simulink model "[6]DPOS_LLC(Matlab2020a)"  (R2020a)
settings: Solver=VariableStepAuto  StartTime=0.0  StopTime=0.01  RelTol=1e-3
libraries: powerlib x24, commsynccomp2 x1, simulink x1
settings Model: Creator=cr  LastModifiedBy=Yatao
settings DataIOCC: ReturnWorkspaceOutputs=off
settings DebuggingCC: ArithmeticOperatorsInVariantConditions=warning
settings SFSimCC: SimUseLocalCustomCode=off  CustomCodeUndefinedFunction=UseInterfaceOnly
settings RTWCC: RTWUseLocalCustomCode=off
settings CodeAppCC: StateflowObjectComments=on
settings SimscapeCC: SimscapeNormalizeSystem=off

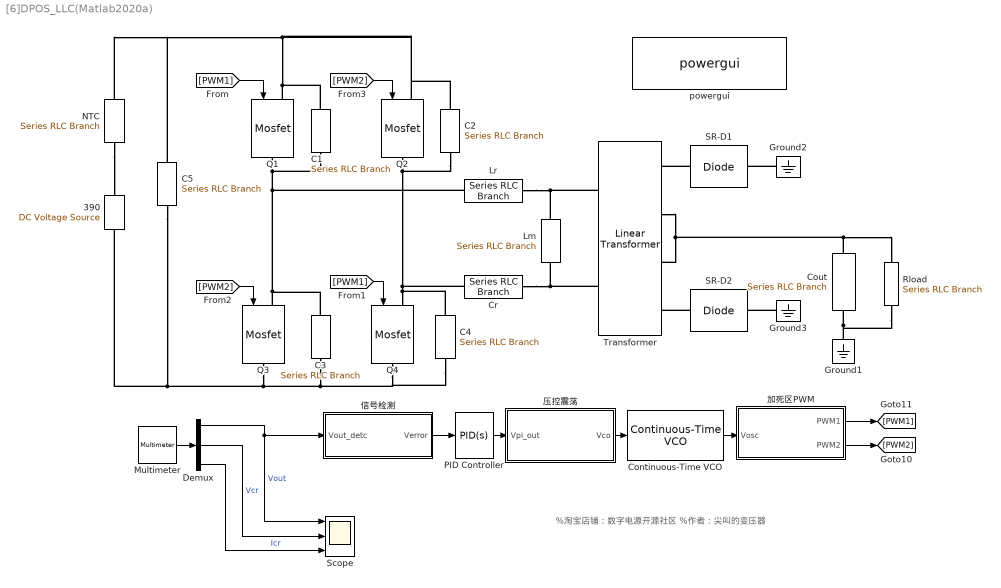
== system [6]DPOS_LLC(Matlab2020a) ==
  note: %淘宝店铺：数字电源开源社区
      | %作者：尖叫的变压器
  " Transformer" : powerlib/Elements/Linear Transformer  UNITS=pu  NominalPower=[ 5000 100e3 ]  winding1=[ 400 0 0 ]  winding2=[ 21 0 0 ]  ThreeWindings=on  winding3=[ 21 0 0 ]  RmLm=[ 1e9 inf ]  Measurements=None  DataType=off
  390 : powerlib/Electrical Sources/DC Voltage Source  Amplitude=390  Measurements=None
  C{1..4} (4 alike) : powerlib/Elements/Series RLC Branch  LConnTagsString=__new0  RConnTagsString=__new0  BranchType=C  Resistance=1  Inductance=1e-3  SetiL0=off  InitialCurrent=0  Capacitance=100e-12  Setx0=off  InitialVoltage=0  Measurements=None
  C5 : powerlib/Elements/Series RLC Branch  LConnTagsString=__new0  RConnTagsString=__new0  BranchType=C  Resistance=1  Inductance=1e-3  SetiL0=off  InitialCurrent=0  Capacitance=100e-6  Setx0=off  InitialVoltage=0  Measurements=None
  Continuous-Time VCO : commsynccomp2/Continuous-Time VCO  Ac=1  Fc=0  Kc=1  Ph=0
      settings: SourceProductBaseCode=CM
  Cout : powerlib/Elements/Series RLC Branch  LConnTagsString=__new0  RConnTagsString=__new0  BranchType=C  Resistance=1  Inductance=1e-3  SetiL0=off  InitialCurrent=0  Capacitance=6000e-6  Setx0=off  InitialVoltage=0  Measurements=None
  Cr : powerlib/Elements/Series RLC Branch  LConnTagsString=__new0  RConnTagsString=__new0  BranchType=C  Resistance=1  Inductance=1e-3  SetiL0=off  InitialCurrent=0  Capacitance=10e-9  Setx0=off  InitialVoltage=0  Measurements=Branch voltage and current
  Demux : Demux  Outputs=3
  Ground1 : powerlib/Elements/Ground  LConnTagsString=a
  Ground2 : powerlib/Elements/Ground  LConnTagsString=a
  Ground3 : powerlib/Elements/Ground  LConnTagsString=a
  Lm : powerlib/Elements/Series RLC Branch  LConnTagsString=__new0  RConnTagsString=__new0  BranchType=L  Resistance=1  Inductance=1500e-6  SetiL0=off  InitialCurrent=0  Capacitance=1e-6  Setx0=off  InitialVoltage=0  Measurements=None
  Lr : powerlib/Elements/Series RLC Branch  LConnTagsString=__new0  RConnTagsString=__new0  BranchType=L  Resistance=1  Inductance=300e-6  SetiL0=off  InitialCurrent=0  Capacitance=1e-6  Setx0=off  InitialVoltage=0  Measurements=None
  Multimeter : powerlib/Measurements/Multimeter  PhasorSimulation=off  OutputType=Complex  sel=[2 1 3]  L=3  Gain=[1 1 1]  yselected={'Ub: Rload','Ub: Cr','Ib: Cr'};  PSBOutputType=1  PSBequivalent=0  AxesSetting=[0,0.1,-100,100]  Display=0  SavedBlockNames=-11
  NTC : powerlib/Elements/Series RLC Branch  LConnTagsString=__new0  RConnTagsString=__new0  BranchType=R  Resistance=1  Inductance=1e-3  SetiL0=off  InitialCurrent=0  Capacitance=100e-12  Setx0=off  InitialVoltage=0  Measurements=None
  PID Controller : simulink/Continuous/PID Controller  Controller=PID  Form=Parallel  TimeDomain=Continuous-time  UseExternalTs=off  SampleTime=-1  IntegratorMethod=Forward Euler  FilterMethod=Forward Euler  ControllerParametersSource=internal  P=0.5  I=0.8  D=2.0  UseFilter=on  N=1  TunerSelectOption=Transfer Function Based (PID Tuner App)  ZeroCross=off  InitialConditionSource=internal  InitialConditionForIntegrator=0  InitialConditionForFilter=0  DifferentiatorICPrevScaledInput=0  ExternalReset=none  TrackingMode=off  Kt=1  LimitOutput=off  UpperSaturationLimit=inf  LowerSaturationLimit=-inf  LinearizeAsGain=on  AntiWindupMode=none  Kb=1  POutMin=[]  POutMax=[]  IOutMin=[]  IOutMax=[]  DOutMin=[]  DOutMax=[]  NOutMin=[]  NOutMax=[]  SumOutMin=[]  SumOutMax=[]  SaturationOutMin=[]  SaturationOutMax=[]  PParamMin=[]  PParamMax=[]  IParamMin=[]  IParamMax=[]  DParamMin=[]  DParamMax=[]  NParamMin=[]  NParamMax=[]  KbParamMin=[]  KbParamMax=[]  KtParamMin=[]  KtParamMax=[]  KbOutMin=[]  KbOutMax=[]  KtOutMin=[]  KtOutMax=[]  IntegratorOutMin=[]  IntegratorOutMax=[]  FilterOutMin=[]  FilterOutMax=[]  SumI1OutMin=[]  SumI1OutMax=[]  SumI2OutMin=[]  SumI2OutMax=[]  SumI3OutMin=[]  SumI3OutMax=[]  SumI4OutMin=[]  SumI4OutMax=[]  SumDOutMin=[]  SumDOutMax=[]  DifferentiatorOutMin=[]  DifferentiatorOutMax=[]  FilterDiffOutCoefMin=[]  FilterDiffOutCoefMax=[]  ReciprocalOutMin=[]  ReciprocalOutMax=[]  SumDenOutMin=[]  SumDenOutMax=[]  SumNumOutMin=[]  SumNumOutMax=[]  DivideOutMin=[]  DivideOutMax=[]  UdiffTsProdOutMin=[]  UdiffTsProdOutMax=[]  NTsProdOutMin=[]  NTsProdOutMax=[]  UintegralTsProdOutMin=[]  UintegralTsProdOutMax=[]  UngainTsProdOutMin=[]  UngainTsProdOutMax=[]  IntegratorContinuousStateAttributes=''  IntegratorStateMustResolveToSignalObject=off  IntegratorRTWStateStorageClass=Auto  FilterContinuousStateAttributes=''  FilterStateMustResolveToSignalObject=off  FilterRTWStateStorageClass=Auto  ParallelPVariant=InternalParameters  IdealPVariant=Disabled  IVariant=InternalParameters  DVariant=InternalParameters  IntegratorVariant=Continuous  SatVariant=Disabled  AWVariant=Passthrough  PCopyVariant=Disabled  TRVariant=Disabled  FdbkBlocksVariant=Forward  IdealPFdbkVariant=Disabled  SatFdbkVariant=Disabled  DerivativeFilterVariant=ContFilter  NVariant=InternalParameters  NCopyVariant=Disabled  FilterICVariant=InternalICsFilter  IntegratorICVariant=InternalICs  ExternalResetVariant=Disabled  TRSumVariant=Passthrough  SumFdbkVariant=Disabled  SumVariant=Sum_PID  TsampFilterVariant=InternalTs  TsampNgainVariant=Passthrough  TsampIntegralVariant=Passthrough
  Q{1..4} (4 alike) : powerlib/Power Electronics/Mosfet  Ron=0.1  Lon=0  Rd=0.07  Vfd=0  IC=0  Rs=1e9  Cs=inf  Measurements=off
  Rload : powerlib/Elements/Series RLC Branch  LConnTagsString=__new0  RConnTagsString=__new0  BranchType=R  Resistance=5  Inductance=1e-3  SetiL0=off  InitialCurrent=0  Capacitance=1e-6  Setx0=off  InitialVoltage=0  Measurements=Branch voltage
  SR-D1 : powerlib/Power Electronics/Diode  Ron=0.001  Lon=0  Vf=0.7  IC=0  UseSnubber=off  Rs=5e9  Cs=10e-12  Measurements=off
  SR-D2 : powerlib/Power Electronics/Diode  Ron=0.001  Lon=0  Vf=0.7  IC=0  UseSnubber=off  Rs=5e9  Cs=10e-12  Measurements=off
  Scope : Scope  NumInputPorts=3
  powergui : powerlib/powergui  Priority=1  SimulationMode=Discrete  SampleTime=1e-8  frequency=60  Iterations=50  frequencyindice=0  Pbase=100e6  ErrMax=1e-4  UnitsV=kV  UnitsW=MW  buscounter=0  FunctionMessages=off  echomessages=off  EnableUseOfTLC=off  CurrentSourceSwitches=off  DisableSnubberDevices=off  DisableRonSwitches=off  DisableVfSwitches=off  DisplayEquations=off  AutomaticDiscreteSolvers=off  SolverType=Tustin/Backward Euler (TBE)  Interpol=off  ExternalGateDelay=off  methode=off  Ts=10  x0status=blocks  SPID=off  SwTol=0  HookPort=off  NonlinearTolerance=1e-4  nMaxIteration=100  ContinueOnMaxIteration=off  RestoreLinks=warning  ResistiveCurrentMeasurement=off  Frange=[0:2:500]  Ylog=off  Xlog=on  ShowGrid=off  save=off  variable=ZData  structure=0  ZoomFFT=off  StartTime=0.0  cycles=1  DisplayStyle=1  fundamental=60  FreqAxis=off  MaxFrequency=1000  frequencyindicesteady=1  RmsSteady=1  display=off
  信号检测 : MATLAB Function  TreatAsAtomicUnit=on
  加死区PWM : MATLAB Function  TreatAsAtomicUnit=on
  压控震荡 : MATLAB Function  TreatAsAtomicUnit=on
  wires:
  [PWM1] -> Q1/1
  [PWM1] -> Q4/1
  [PWM2] -> Q3/1
  [PWM2] -> Q2/1
  信号检测/1(Verror) -> PID Controller/1
  Continuous-Time VCO/1 -> 加死区PWM/1(Vosc)
  加死区PWM/1(PWM1) -> [PWM1]
  加死区PWM/2(PWM2) -> [PWM2]
  压控震荡/1(Vco) -> Continuous-Time VCO/1
  PID Controller/1 -> 压控震荡/1(Vpi_out)
  Multimeter/1 -> Demux/1
  Demux/1 -> Scope/1, 信号检测/1(Vout_detc)  "Vout"
  Demux/2 -> Scope/2  "Vcr"
  Demux/3 -> Scope/3  "Icr"
  connections:
  C3/RConn1 -- C4/RConn1 -- Q4/RConn1 -- Q3/RConn1 -- 390/LConn1 -- C5/RConn1
  C1/LConn1 -- C5/LConn1 -- NTC/LConn1 -- C2/LConn1 -- Q2/LConn1 -- Q1/LConn1
  Q3/LConn1 -- C3/LConn1 -- C1/RConn1 -- Q1/RConn1 -- Lr/RConn1
  Q2/RConn1 -- C2/RConn1 -- Cr/LConn1 -- C4/LConn1 -- Q4/LConn1
  " Transformer"/LConn1 -- Lr/LConn1 -- Lm/RConn1
  Cout/LConn1 -- Rload/LConn1 -- " Transformer"/RConn2 -- " Transformer"/RConn3
  Rload/RConn1 -- Ground1/LConn1 -- Cout/RConn1
  SR-D1/RConn1 -- " Transformer"/RConn1
  SR-D2/RConn1 -- " Transformer"/RConn4
  Ground2/LConn1 -- SR-D1/LConn1
  Ground3/LConn1 -- SR-D2/LConn1
  " Transformer"/LConn2 -- Cr/RConn1 -- Lm/LConn1
  NTC/RConn1 -- 390/RConn1

== matlab function [6]DPOS_LLC(Matlab2020a)/信号检测 ==
  data: Vout_detc input; Verror output
function Verror  = fcn(Vout_detc)
Verror=21-Vout_detc;
%作者：尖叫的变压器
%淘宝店铺：数字电源开源社区

== matlab function [6]DPOS_LLC(Matlab2020a)/加死区PWM ==
  data: Vosc input; PWM1 output; PWM2 output
function [PWM1,PWM2]  = fcn(Vosc)
if(Vosc>0.1)
    PWM1=12;
else
    PWM1=0;
end

if(-Vosc>0.1)
    PWM2=12;
else
    PWM2=0;
end

%作者：尖叫的变压器
%淘宝店铺：数字电源开源社区

== matlab function [6]DPOS_LLC(Matlab2020a)/压控震荡 ==
  data: Vpi_out input; Vco output
function Vco   = fcn(Vpi_out)
if(Vpi_out>3.3)
    Vpi_out=3.3;
end
if(Vpi_out<0)
    Vpi_out=0;
end
%我们希望误差电压越大频率越低。
%即（0,65KHz），（3.3,300KHz）
k=-(300*10^3-65*10^3)/3.3;
Vco=Vpi_out*k+300*10^3;
%作者：尖叫的变压器
%淘宝店铺：数字电源开源社区
